simulink library "INT_DevLib_PwrStgState"  (R2016b)
settings: Solver=VariableStepAuto  StartTime=0.0  StopTime=10.0  RelTol=1e-3
settings Model: Creator=Administrator  LastModifiedBy=Administrator

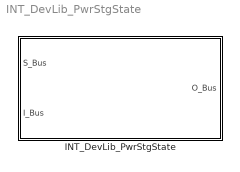
== system INT_DevLib_PwrStgState ==
  INT_DevLib_PwrStgState : Subsystem

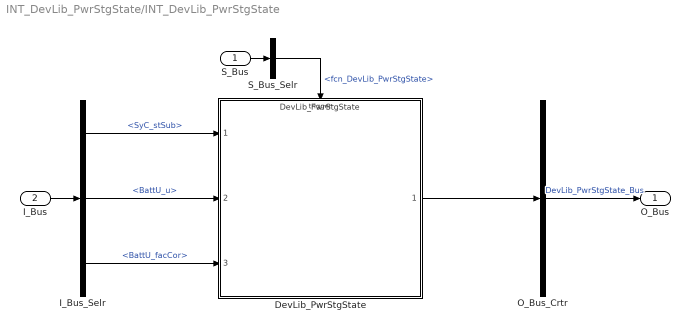
== system INT_DevLib_PwrStgState/INT_DevLib_PwrStgState ==
  S_Bus : Inport
  I_Bus : Inport  Port=2
  DevLib_PwrStgState : ModelReference  ModelNameDialog=DevLib_PwrStgState  SimulationMode=Normal  ModelReferenceVersion=1.5  TriggerPortName=function  TriggerPortTriggerType=function-call  TriggerPortStatesWhenEnabling=held
  I_Bus_Selr : BusSelector  OutputSignals=SyC_stSub,BattU_u,BattU_facCor
  O_Bus_Crtr : BusCreator  Inputs=1
  S_Bus_Selr : BusSelector  OutputSignals=fcn_DevLib_PwrStgState
  O_Bus : Outport
  wires:
  S_Bus_Selr/1 -> DevLib_PwrStgState/Trigger  "<fcn_DevLib_PwrStgState>"
  S_Bus/1 -> S_Bus_Selr/1
  I_Bus/1 -> I_Bus_Selr/1
  I_Bus_Selr/1 -> DevLib_PwrStgState/1  "<SyC_stSub>"
  I_Bus_Selr/2 -> DevLib_PwrStgState/2  "<BattU_u>"
  I_Bus_Selr/3 -> DevLib_PwrStgState/3  "<BattU_facCor>"
  O_Bus_Crtr/1 -> O_Bus/1  "DevLib_PwrStgState_Bus"
  DevLib_PwrStgState/1 -> O_Bus_Crtr/1
